simulink model "Subsistema_termico"  (R2021a)
settings: Solver=VariableStepAuto  StartTime=0.0  StopTime=10.0  RelTol=1e-3
undefined symbols (not defined in the file): alpha_cu, Cts, Rs_REF, Rts_amb, Ts_REF
settings Model: Creator=fhlla  LastModifiedBy=fhlla

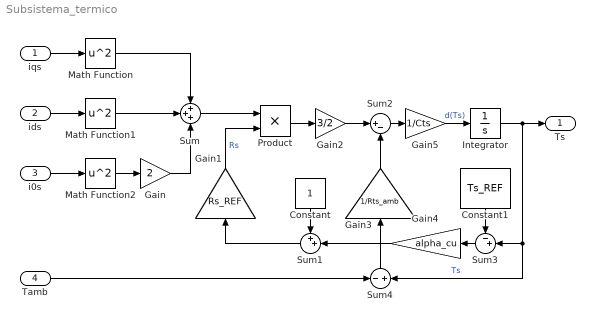
== system Subsistema_termico ==
  iqs : Inport
  ids : Inport  Port=2
  i0s : Inport  Port=3
  Tamb : Inport  Port=4
  Constant : Constant
  Constant1 : Constant  Value=Ts_REF
  Gain : Gain  Gain=2
  Gain1 : Gain  Gain=Rs_REF
  Gain2 : Gain  Gain=3/2
  Gain3 : Gain  Gain=1/Rts_amb
  Gain4 : Gain  Gain=alpha_cu
  Gain5 : Gain  Gain=1/Cts
  Integrator : Integrator
  Math Function : Math  Operator=square  SaturateOnIntegerOverflow=on
  Math Function1 : Math  Operator=square  SaturateOnIntegerOverflow=on
  Math Function2 : Math  Operator=square  SaturateOnIntegerOverflow=on
  Product : Product
  Sum : Sum  Inputs=+++
  Sum1 : Sum  Inputs=++|
  Sum2 : Sum  Inputs=|+-
  Sum3 : Sum  Inputs=-+|
  Sum4 : Sum  Inputs=-|+
  Ts : Outport
  wires:
  Math Function2/1 -> Gain/1
  Gain2/1 -> Sum2/1
  Constant/1 -> Sum1/1
  Sum2/1 -> Gain5/1
  Gain5/1 -> Integrator/1  "d(Ts)"
  iqs/1 -> Math Function/1
  ids/1 -> Math Function1/1
  i0s/1 -> Math Function2/1
  Tamb/1 -> Sum4/1
  Sum/1 -> Product/1
  Gain1/1 -> Product/2  "Rs"
  Product/1 -> Gain2/1
  Integrator/1 -> Sum3/2, Sum4/2, Ts/1  "Ts"
  Sum1/1 -> Gain1/1
  Gain4/1 -> Sum1/2
  Sum3/1 -> Gain4/1
  Constant1/1 -> Sum3/1
  Sum4/1 -> Gain3/1
  Gain3/1 -> Sum2/2
  Math Function1/1 -> Sum/2
  Math Function/1 -> Sum/1
  Gain/1 -> Sum/3
